simulink model "Problem4_MotorPositionControl"  (R2020b)
settings: Solver=VariableStepAuto  StartTime=0.0  StopTime=0.4  RelTol=1e-3
undefined symbols (not defined in the file): b, J, K, L, R
settings Model: DataDictionary=Data.sldd  Creator=vigne  LastModifiedBy=znome

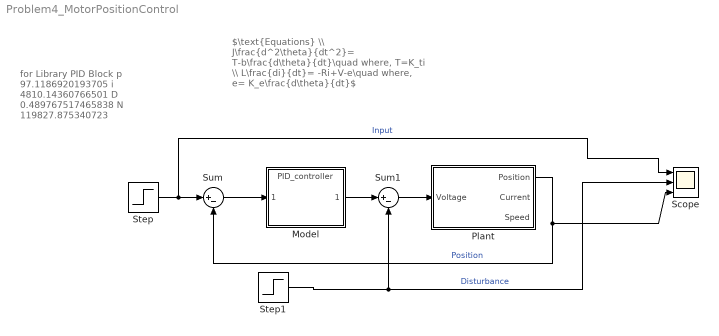
== system Problem4_MotorPositionControl ==
  note: for Library PID Block
      | p 97.1186920193705
      | i 4810.14360766501
      | D 0.489767517465838
      | N 119827.875340723
  note: $\text{Equations} \\ J\frac{d^2\theta}{dt^2}= T-b\frac{d\theta}{dt}\quad where, T=K_ti \\ L\frac{di}{dt}= -Ri+V-e\quad where, e= K_e\frac{d\theta}{dt}$
  Model : ModelReference  ModelNameDialog=PID_controller.slx  SimulationMode=Normal  ModelReferenceVersion=1.4
  Plant : Subsystem
  Scope : Scope  NumInputPorts=3
  Step : Step  Time=0.2  SampleTime=0
  Step1 : Step  Time=0.3  SampleTime=0
  Sum : Sum  Inputs=|+-
  Sum1 : Sum  Inputs=|+-
  wires:
  Plant/1(Position) -> Sum/2, Scope/3  "Position"
  Sum/1 -> Model/1
  Step/1 -> Scope/1, Sum/1  "Input"
  Step1/1 -> Sum1/2, Scope/2  "Disturbance"
  Model/1 -> Sum1/1
  Sum1/1 -> Plant/1(Voltage)

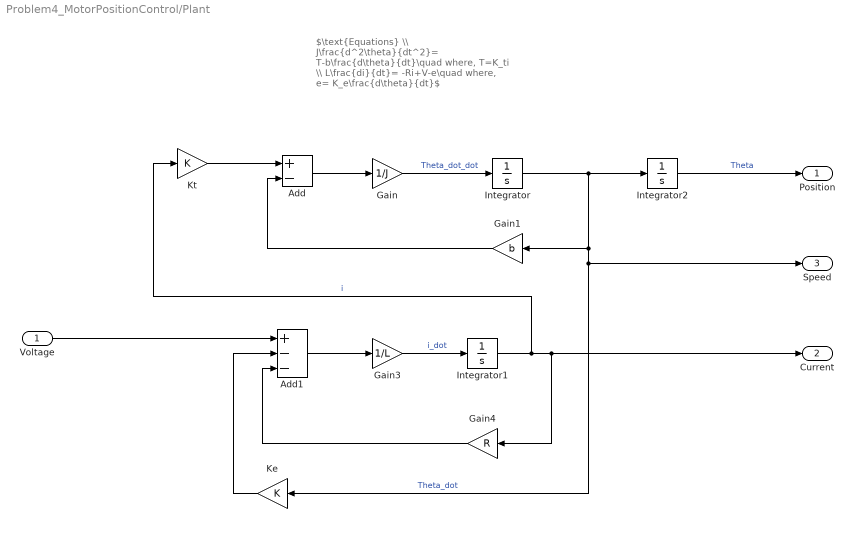
== system Problem4_MotorPositionControl/Plant ==
  note: $\text{Equations} \\ J\frac{d^2\theta}{dt^2}= T-b\frac{d\theta}{dt}\quad where, T=K_ti \\ L\frac{di}{dt}= -Ri+V-e\quad where, e= K_e\frac{d\theta}{dt}$
  Voltage : Inport
  Add : Sum  Inputs=+-
  Add1 : Sum  Inputs=+--
  Gain : Gain  Gain=1/J
  Gain1 : Gain  Gain=b
  Gain3 : Gain  Gain=1/L
  Gain4 : Gain  Gain=R
  Integrator : Integrator
  Integrator1 : Integrator
  Integrator2 : Integrator
  Ke : Gain  Gain=K
  Kt : Gain  Gain=K
  Position : Outport
  Current : Outport  Port=2
  Speed : Outport  Port=3
  wires:
  Integrator/1 -> Integrator2/1, Ke/1, Speed/1, Gain1/1  "Theta_dot"
  Ke/1 -> Add1/2
  Gain1/1 -> Add/2
  Integrator2/1 -> Position/1  "Theta"
  Kt/1 -> Add/1
  Integrator1/1 -> Kt/1, Current/1, Gain4/1  "i"
  Gain4/1 -> Add1/3
  Gain/1 -> Integrator/1  "Theta_dot_dot"
  Add1/1 -> Gain3/1
  Gain3/1 -> Integrator1/1  "i_dot"
  Add/1 -> Gain/1
  Voltage/1 -> Add1/1
